simulink model "Model33"  (R2020a)
settings: Solver=ode45  StartTime=0.0  StopTime=25  MaxStep=0.01  RelTol=1e-3  AbsTol=1e-6
values from neighbouring files (symbols this model uses):
  ctrl = 1.0    [ABSdd.sldd]
  g = 32.18    [ABSdd.sldd]
  m = 50.0    [ABSdd.sldd]
  mu = 0.0 0.4 0.8 0.97 1.0 0.98 0.96 0.94 0.92 0.9 0.88 0.855 0.83 0.81 0.79 0.77 0.75 0.73 0.72 0.71 0.7    [ABSdd.sldd]
  Rr = 1.25    [ABSdd.sldd]
  slip = 0.0 0.05 0.1 0.15000000000000002 0.2 0.25 0.30000000000000004 0.35000000000000003 0.4 0.45 0.5 0.55 0.6 0.64999999999999991 0.7 0.75 0.8 0.85 0.9 0.95 1.0    [ABSdd.sldd]
  v0 = 88.0    [ABSdd.sldd]
settings Model: DataDictionary=ABSdd.sldd  Creator=HP  LastModifiedBy=HP

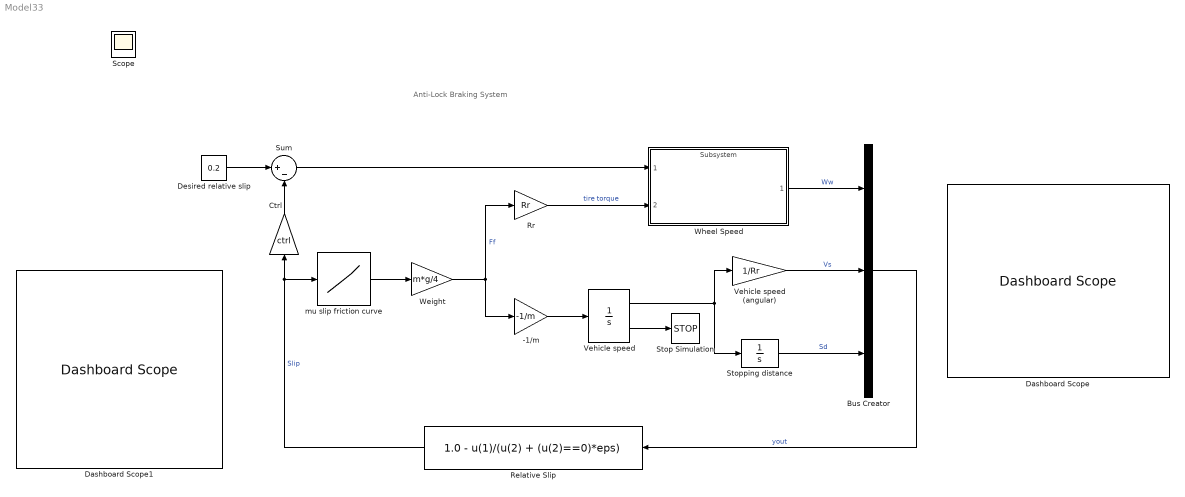
== system Model33 ==
  note: Anti-Lock Braking System
  -1/m : Gain  Gain=-1/m  SaturateOnIntegerOverflow=on  OutDataTypeStr=Inherit: Same as input  ParamDataTypeStr=Inherit: Same as input
  Bus Creator : BusCreator  Inputs=3
  Ctrl : Gain  Gain=ctrl  SaturateOnIntegerOverflow=on  OutDataTypeStr=Inherit: Same as input  ParamDataTypeStr=Inherit: Same as input
  Dashboard Scope : DashboardScope
  Dashboard Scope1 : DashboardScope
  Desired relative slip : Constant  Value=0.2
  Relative Slip : Fcn  Expr=1.0 - u(1)/(u(2) + (u(2)==0)*eps)
  Rr : Gain  Gain=Rr  SaturateOnIntegerOverflow=on  OutDataTypeStr=Inherit: Same as input  ParamDataTypeStr=Inherit: Same as input
  Stop Simulation : Stop
  Stopping distance : Integrator  UpperSaturationLimit=1000  LowerSaturationLimit=0
  Sum : Sum  Inputs=|+-
  Vehicle speed : Integrator  InitialCondition=v0  LimitOutput=on  UpperSaturationLimit=1000  LowerSaturationLimit=0  ShowSaturationPort=on
  "Vehicle speed (angular) " : Gain  Gain=1/Rr  SaturateOnIntegerOverflow=on  OutDataTypeStr=Inherit: Same as input  ParamDataTypeStr=Inherit: Same as input
  Weight : Gain  Gain=m*g/4  SaturateOnIntegerOverflow=on  OutDataTypeStr=Inherit: Same as input  ParamDataTypeStr=Inherit: Same as input
  Wheel Speed : ModelReference  ModelNameDialog=Subsystem  ModelReferenceVersion=1.5
  mu slip friction curve : Lookup_n-D  NumberOfTableDimensions=1  BreakpointsForDimension1=slip  Table=mu  SaturateOnIntegerOverflow=on  InputSameDT=on
  Scope : Scope
  wires:
  Desired relative slip/1 -> Sum/1
  Sum/1 -> Wheel Speed/1
  Ctrl/1 -> Sum/2
  mu slip friction curve/1 -> Weight/1
  Weight/1 -> -1/m/1, Rr/1  "Ff"
  Rr/1 -> Wheel Speed/2  "tire torque"
  -1/m/1 -> Vehicle speed/1
  Vehicle speed/2 -> Stop Simulation/1
  Vehicle speed/1 -> Stopping distance/1, "Vehicle speed (angular) "/1
  Stopping distance/1 -> Bus Creator/3  "Sd"
  "Vehicle speed (angular) "/1 -> Bus Creator/2  "Vs"
  Relative Slip/1 -> mu slip friction curve/1, Ctrl/1  "Slip"
  Wheel Speed/1 -> Bus Creator/1  "Ww"
  Bus Creator/1 -> Relative Slip/1  "yout"
